simulink model "AM_DSB_SC_rxBC"  (R2024b)
settings: Solver=VariableStepAuto  StartTime=0.0  StopTime=inf  RelTol=1e-3
undefined symbols (not defined in the file): Bn, d, fs, Ko, Kp
libraries: dspsrcs4 x4, dspmlti4 x3, dspsnks4 x1, rtlsdr_book_library x1, dspfdesign x1, dspvision x1
settings Model: Creator=javier.alonsov  LastModifiedBy=javier.alonsov

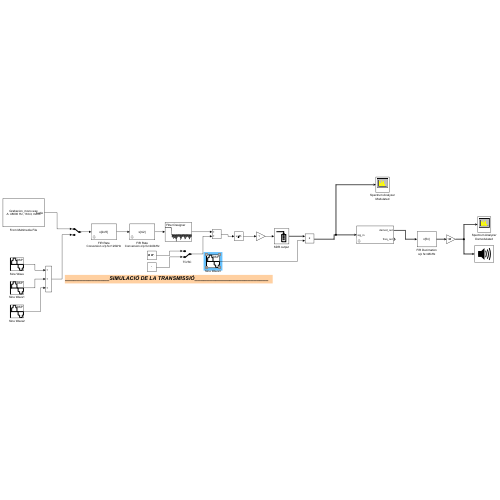
[thumbnail: Simulink's stored preview of the top-level diagram]
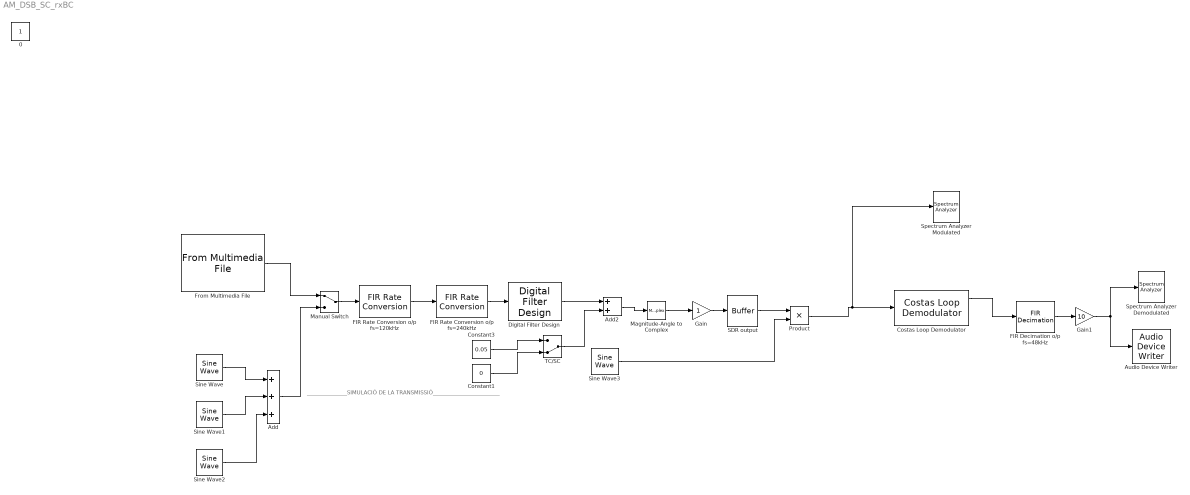
== system AM_DSB_SC_rxBC ==
  note: _______________SIMULACIÓ DE LA TRANSMISSIÓ_________________________
  Add : Sum  Inputs=+++
  Add2 : Sum
  Audio Device Writer : dspsnks4/Audio Device Writer  Driver=DirectSound  Device=Default  InheritSampleRate=on  SampleRate=44100  BitDepth=16-bit integer  BufferSize=4096  NumBuffers=10  DefaultOutputChannelMapping=on  OutputChannelMapping=1:2  OutputNumUnderrunSamples=off  DriverIdx=1  DeviceWarnFlag=''
  Constant1 : Constant  Value=0
  Constant3 : Constant  Value=0.05
  Costas Loop Demodulator : rtlsdr_book_library/Sync Tools for Analogue Comms/Costas Loop Demodulator  filter_type=Type 2  K1_param=(4*d*Bn*1/fs)/(Ko*Kp*(d+1/(4*d)))  K2_param=(4*(Bn*1/fs)^2)/(Ko*Kp*(d+1/4*d)^2)  fs=240e3  fq=40e3  Bn=1e3  d=0.707  frm_size=4096
      settings: SourceProductName=RTL-SDR Book Library
  Digital Filter Design : dspfdesign/Digital Filter Design  mwdsp_browser_bugfix_var=off
  FIR Decimation o/p fs=48kHz : dspmlti4/FIR Decimation  FilterSource=Dialog parameters  h=firpm(200, [0 15e3 20e3 (240e3/2)]/(240e3/2), [1 1 0 0], [1 1], 20)  D=5  filtStruct=Direct form  FilterObject=Hm_firdecim  InputProcessing=Columns as channels (frame based)  framing=Allow multirate processing  AllowArbitraryInputLength=off  inputOffset=0  outputBufInitCond=0  roundingMode=Floor  overflowMode=off  firstCoeffDataTypeStr=Inherit: Same word length as input  firstCoeffMin=[]  firstCoeffMax=[]  firstCoeffLastDataTypeStr=Inherit: Same word length as input  outputDataTypeStr=Inherit: Same as accumulator  outputMin=[]  outputMax=[]  outputLastDataTypeStr=Inherit: Same as accumulator
  FIR Rate Conversion o/p fs=120kHz : dspmlti4/FIR Rate Conversion  FilterSource=Dialog parameters  L=5  h=firpm(50,[0 15e3 24e3 240e3/2]/(240e3/2),[1 1 0 0], [1 1],20)  M=2  FilterObject=FRC  rateMode=Enforce single-rate processing  AllowArbitraryInputLength=off  roundingMode=Floor  overflowMode=off  firstCoeffDataTypeStr=Inherit: Same word length as input  firstCoeffMin=[]  firstCoeffMax=[]  firstCoeffLastDataTypeStr=Inherit: Same word length as input  outputDataTypeStr=Inherit: Same as accumulator  outputMin=[]  outputMax=[]  outputLastDataTypeStr=Inherit: Same as accumulator
  FIR Rate Conversion o/p fs=240kHz : dspmlti4/FIR Rate Conversion  FilterSource=Auto  L=2  h=firpm(50,[0 15e3 30e3 600e3/2]/(600e3/2),[1 1 0 0], [1 1],20)  M=1  FilterObject=FRC  rateMode=Allow multirate processing  AllowArbitraryInputLength=off  roundingMode=Floor  overflowMode=off  firstCoeffDataTypeStr=Inherit: Same word length as input  firstCoeffMin=[]  firstCoeffMax=[]  firstCoeffLastDataTypeStr=Inherit: Same word length as input  outputDataTypeStr=Inherit: Same as accumulator  outputMin=[]  outputMax=[]  outputLastDataTypeStr=Inherit: Same as accumulator
  From Multimedia File : dspvision/From Multimedia File  inputFilename=C:\Users\javier.alonsov\Documents\Curso25_26\Docencia\GET\SISCOM\LAB\SDR_3_DesmodAMNoCoherent\Grabacion_mono.wav  readRange=[1 Inf]  loop=on  numPlays=inf  outputStreams=Audio only  videoDataType=single  audioDataType=single  inheritSampleTime=on  userDefinedSampleTime=1/30  noAudioOutput=off  isIntensityVideo=off  fourcc=RGB  colorVideoFormat=One multidimensional signal  outputEOF=off  dataOrg=Column-major  audioFrameSize=600  computeAudioFrameSize=off  outSamplingMode=Sample based
      settings: LibrarySourceBlock=dspsrcs4/From Multimedia File
  Gain : Gain
  Gain1 : Gain  Gain=10
  Magnitude-Angle to Complex : MagnitudeAngleToComplex  Input=Magnitude
  Manual Switch : ManualSwitch
  Product : Product
  SDR output : Buffer  N=4096
  Sine Wave : dspsrcs4/Sine Wave  Amplitude=0.05  Frequency=1e3  Phase=0  SampleMode=Discrete  OutComplex=Real  CompMethod=Trigonometric fcn  TableSize=Speed  SampleTime=1/48e3  SamplesPerFrame=600  ResetState=Restart at time zero  OutputFrames=off  dataType=double  wordLen=16  udDataType=sfix(16)  fracBitsMode=Best precision  numFracBits=15  OutDataTypeStr=double  LastOutDataTypeStr=double
  Sine Wave1 : dspsrcs4/Sine Wave  Amplitude=0.05  Frequency=5e3  Phase=0  SampleMode=Discrete  OutComplex=Real  CompMethod=Trigonometric fcn  TableSize=Speed  SampleTime=1/48e3  SamplesPerFrame=600  ResetState=Restart at time zero  OutputFrames=off  dataType=double  wordLen=16  udDataType=sfix(16)  fracBitsMode=Best precision  numFracBits=15  OutDataTypeStr=double  LastOutDataTypeStr=double
  Sine Wave2 : dspsrcs4/Sine Wave  Amplitude=0.05  Frequency=10e3  Phase=0  SampleMode=Discrete  OutComplex=Real  CompMethod=Trigonometric fcn  TableSize=Speed  SampleTime=1/48e3  SamplesPerFrame=600  ResetState=Restart at time zero  OutputFrames=off  dataType=double  wordLen=16  udDataType=sfix(16)  fracBitsMode=Best precision  numFracBits=15  OutDataTypeStr=double  LastOutDataTypeStr=double
  Sine Wave3 : dspsrcs4/Sine Wave  Amplitude=1  Frequency=39.6e3  Phase=0  SampleMode=Discrete  OutComplex=Complex  CompMethod=Trigonometric fcn  TableSize=Speed  SampleTime=1/240e3  SamplesPerFrame=4096  ResetState=Restart at time zero  OutputFrames=off  dataType=double  wordLen=16  udDataType=sfix(16)  fracBitsMode=Best precision  numFracBits=15  OutDataTypeStr=double  LastOutDataTypeStr=double
  Spectrum Analyzer Demodulated : SpectrumAnalyzer  WindowPosition=[1.000000,49.000000,1920.000000,1009.000000,]  Visible=on  ScopeFrameLocation=window  Method=Welch  SampleRate=48000  AxesScaling=Manual  Span=240000  StartFrequency=-120000  StopFrequency=120000  AveragingMethod=Running  YLimits=[-180.94415229593105,48.14480110113395]  AllowFFTLengthLessThanSamplesPerUpdate=on  DefaultConfigurationName=spbscopes.SpectrumAnalyzerBlockCfg  IsFrequencyInputMode=0  FrequencyVectorPort=0  FrequencyVectorFromPort=0  FrequencyInputRBWPort=0  FrequencyInputRBWFromPort=0
  Spectrum Analyzer Modulated : SpectrumAnalyzer  WindowPosition=[1070.000000,261.000000,777.000000,407.000000,]  Visible=on  ScopeFrameLocation=window  Method=Welch  SampleRate=240000  AxesScaling=Manual  Span=240000  StartFrequency=-120000  StopFrequency=120000  AveragingMethod=Running  YLimits=[-278.33171856834804,158.35436536760395]  AllowFFTLengthLessThanSamplesPerUpdate=on  DefaultConfigurationName=spbscopes.SpectrumAnalyzerBlockCfg  IsFrequencyInputMode=0  FrequencyVectorPort=0  FrequencyVectorFromPort=0  FrequencyInputRBWPort=0  FrequencyInputRBWFromPort=0
  TC/SC : ManualSwitch  CurrentSetting=0
  0 : Constant  IOType=siggen
  wires:
  FIR Rate Conversion o/p fs=120kHz/1 -> FIR Rate Conversion o/p fs=240kHz/1
  Manual Switch/1 -> FIR Rate Conversion o/p fs=120kHz/1
  From Multimedia File/1 -> Manual Switch/1
  Sine Wave/1 -> Add/1
  Sine Wave1/1 -> Add/2
  Sine Wave2/1 -> Add/3
  Add/1 -> Manual Switch/2
  FIR Rate Conversion o/p fs=240kHz/1 -> Digital Filter Design/1
  Digital Filter Design/1 -> Add2/1
  Magnitude-Angle to Complex/1 -> Gain/1
  FIR Decimation o/p fs=48kHz/1 -> Gain1/1
  Constant3/1 -> TC/SC/1
  TC/SC/1 -> Add2/2
  Constant1/1 -> TC/SC/2
  Costas Loop Demodulator/1 -> FIR Decimation o/p fs=48kHz/1
  Gain1/1 -> Audio Device Writer/1, Spectrum Analyzer Demodulated/1
  Gain/1 -> SDR output/1
  Add2/1 -> Magnitude-Angle to Complex/1
  SDR output/1 -> Product/1
  Sine Wave3/1 -> Product/2
  Product/1 -> Spectrum Analyzer Modulated/1, Costas Loop Demodulator/1
